simulink model "week2model"  (R2026a)
settings: Solver=VariableStepAuto  StopTime=0.5
model workspace (MAT data in the model file):
  Kp = 0.05
settings Model: Creator=michaeljohansen  LastModifiedBy=michaeljohansen

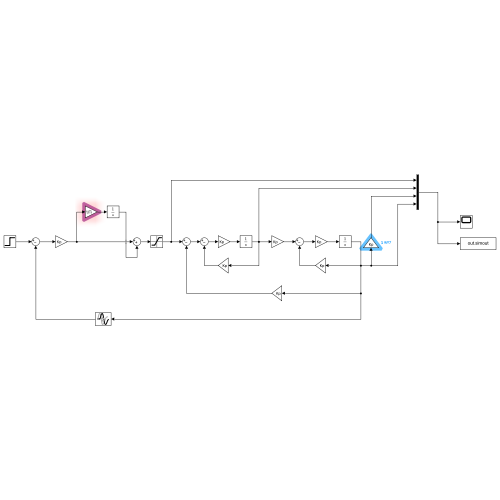
[thumbnail: Simulink's stored preview of the top-level diagram]
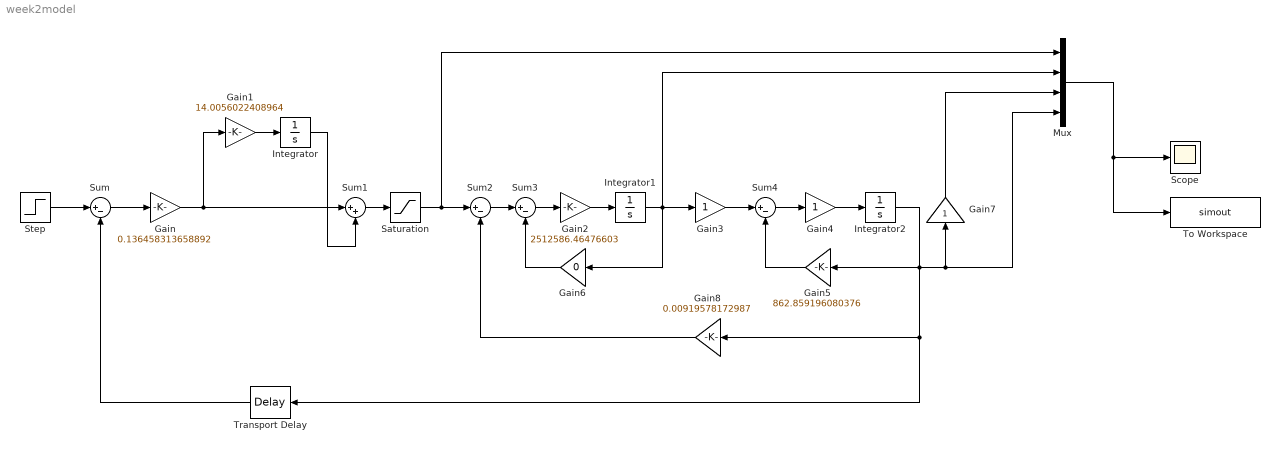
== system week2model ==
  Gain : Gain  Gain=0.136458313658892
  Gain1 : Gain  Gain=14.0056022408964
  Gain2 : Gain  Gain=2512586.46476603
  Gain3 : Gain  Gain=1
  Gain4 : Gain  Gain=1
  Gain5 : Gain  Gain=862.859196080376
  Gain6 : Gain  Gain=0
  Gain7 : Gain  Gain=1
  Gain8 : Gain  Gain=0.00919578172987
  Integrator : Integrator
  Integrator1 : Integrator
  Integrator2 : Integrator
  Mux : Mux
  Saturation : Saturate
  Scope : Scope
  Step : Step  SampleTime=0
  Sum{,2..4} (4 alike) : Sum  Inputs=|+-
  Sum1 : Sum  Inputs=|++
  To Workspace : ToWorkspace  VariableName=simout  SaveFormat=Timeseries  SampleTime=-1
  Transport Delay : TransportDelay  DelayTime=0.01
  wires:
  Step/1 -> Sum/1
  Sum/1 -> Gain/1
  Gain1/1 -> Integrator/1
  Gain/1 -> Gain1/1, Sum1/1
  Integrator/1 -> Sum1/2
  Sum1/1 -> Saturation/1
  Transport Delay/1 -> Sum/2
  Saturation/1 -> Mux/1, Sum2/1
  Sum2/1 -> Sum3/1
  Sum3/1 -> Gain2/1
  Gain2/1 -> Integrator1/1
  Integrator1/1 -> Mux/2, Gain6/1, Gain3/1
  Gain3/1 -> Sum4/1
  Gain4/1 -> Integrator2/1
  Integrator2/1 -> Mux/4, Gain7/1, Gain5/1, Transport Delay/1, Gain8/1
  Gain5/1 -> Sum4/2
  Gain6/1 -> Sum3/2
  Sum4/1 -> Gain4/1
  Gain8/1 -> Sum2/2
  Gain7/1 -> Mux/3
  Mux/1 -> Scope/1, To Workspace/1
